simulink subsystem "visualization"  (R2025b)
settings: Solver=VariableStepAuto  StartTime=0.0  StopTime=10.0  RelTol=1e-3
undefined symbols (not defined in the file): alt, angle_vert_deg, crossrange, location, sim_time, vel_ver
libraries: aerolibanim x1, simulink_extras x1
settings Model: Creator=joedo  LastModifiedBy=finnb

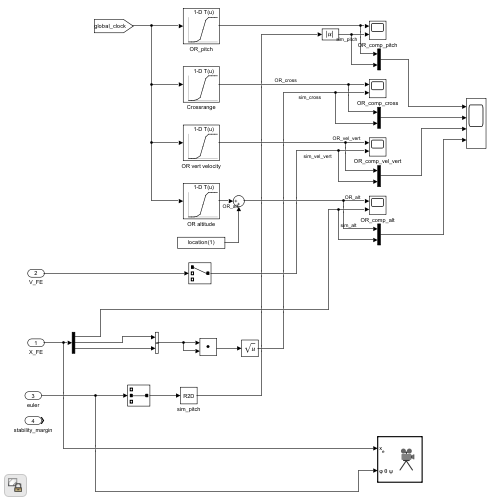
[thumbnail: Simulink's stored preview of the top-level diagram]
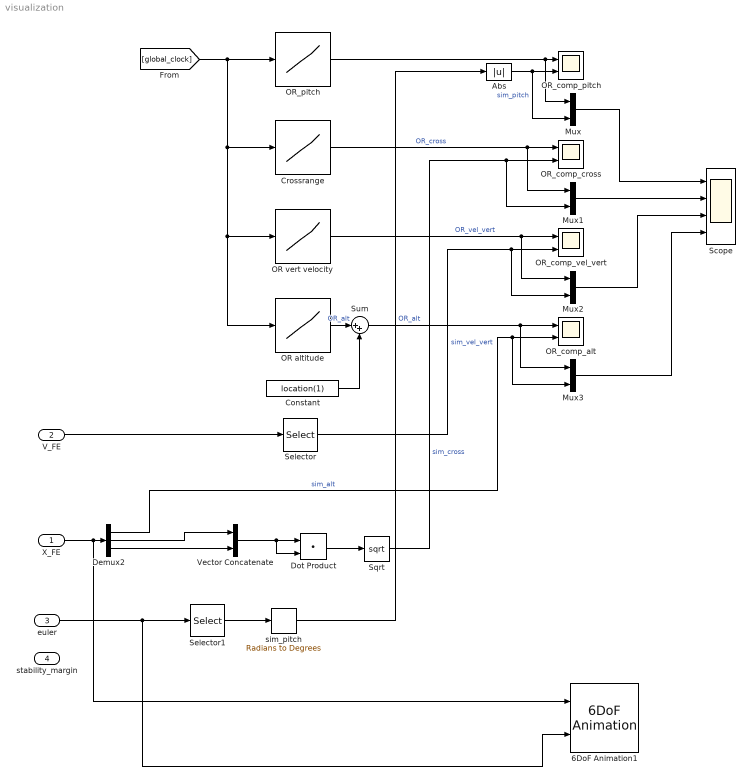
== system visualization ==
  X_FE : Inport
  V_FE : Inport  Port=2
  euler : Inport  Port=3
  stability_margin : Inport  Port=4
  6DoF Animation1 : aerolibanim/6DoF Animation  u1=[0 8000 -100 100 0 400]  u2=0.1  u3=5  u4=[location(1)-5 0 0]  u5=Fly alongside  u6=[-50 20 0]  u7=10  u8=off
  Abs : Abs  SaturateOnIntegerOverflow=off
  Constant : Constant  Value=location(1)
  Crossrange : Lookup_n-D  NumberOfTableDimensions=1  BreakpointsForDimension1=sim_time  Table=crossrange  InternalRulePriority=Speed  RndMeth=Simplest
  Demux2 : Demux  Outputs=3
  Dot Product : DotProduct  OutDataTypeStr=Inherit: Inherit via internal rule
  Mux{,1..3} (4 alike) : Mux  Inputs=2
  OR altitude : Lookup_n-D  NumberOfTableDimensions=1  BreakpointsForDimension1=sim_time  Table=alt  InternalRulePriority=Speed  RndMeth=Simplest
  OR vert velocity : Lookup_n-D  NumberOfTableDimensions=1  BreakpointsForDimension1=sim_time  Table=vel_ver  InternalRulePriority=Speed  RndMeth=Simplest
  OR_comp_alt : Scope  NumInputPorts=2
      settings: ActiveDisplayYMinimum=-838.88766  ActiveDisplayYMaximum=7549.94141  DataLoggingVariableName=ScopeData5
  OR_comp_cross : Scope  NumInputPorts=2
      settings: ActiveDisplayYMinimum=-199.36184  ActiveDisplayYMaximum=1794.25654  DataLoggingVariableName=ScopeData6
  OR_comp_pitch : Scope  NumInputPorts=2
      settings: ActiveDisplayYMinimum=-13.012  ActiveDisplayYMaximum=167.10802  DataLoggingVariableName=ScopeData14
  OR_comp_vel_vert : Scope  NumInputPorts=2
      settings: ActiveDisplayYMinimum=-95.80315  ActiveDisplayYMaximum=488.12758  DataLoggingVariableName=ScopeData15
  OR_pitch : Lookup_n-D  NumberOfTableDimensions=1  BreakpointsForDimension1=sim_time  Table=angle_vert_deg  InternalRulePriority=Speed  RndMeth=Simplest
  Scope : Scope  NumInputPorts=4
      settings: ActiveDisplayYMinimum=-5.57011622160341  ActiveDisplayYMaximum=50.131045994430721  DataLoggingVariableName=ScopeData9
  Selector : Selector  InputPortWidth=3  IndexOptions=Index vector (dialog)  Indices=[1]  OutputSizes=1
  Selector1 : Selector  InputPortWidth=3  IndexOptions=Index vector (dialog)  Indices=[2]  OutputSizes=1
  Sqrt : Sqrt
  Sum : Sum  Inputs=|++
  Vector Concatenate : Concatenate
  sim_pitch : simulink_extras/Transformations/Radians to Degrees
  wires:
  Vector Concatenate/1 -> Dot Product/1, Dot Product/2
  Demux2/2 -> Vector Concatenate/1
  Crossrange/1 -> Mux1/1, OR_comp_cross/1  "OR_cross"
  [global_clock] -> OR_pitch/1, OR altitude/1, OR vert velocity/1, Crossrange/1
  Demux2/3 -> Vector Concatenate/2
  OR_pitch/1 -> Mux/1, OR_comp_pitch/1
  Selector1/1 -> sim_pitch/1
  sim_pitch/1 -> Abs/1
  Sum/1 -> Mux3/1, OR_comp_alt/1  "OR_alt"
  Demux2/1 -> OR_comp_alt/2, Mux3/2  "sim_alt"
  Selector/1 -> OR_comp_vel_vert/2, Mux2/2  "sim_vel_vert"
  Dot Product/1 -> Sqrt/1
  Sqrt/1 -> OR_comp_cross/2, Mux1/2  "sim_cross"
  OR vert velocity/1 -> OR_comp_vel_vert/1, Mux2/1  "OR_vel_vert"
  V_FE/1 -> Selector/1
  Abs/1 -> Mux/2, OR_comp_pitch/2  "sim_pitch"
  Mux/1 -> Scope/1
  Mux1/1 -> Scope/2
  Mux2/1 -> Scope/3
  Mux3/1 -> Scope/4
  OR altitude/1 -> Sum/1  "OR_alt"
  Constant/1 -> Sum/2
  X_FE/1 -> Demux2/1, 6DoF Animation1/1
  euler/1 -> Selector1/1, 6DoF Animation1/2
